simulink library "Controller_Lib"  (Simulink 8.4)
settings: Solver=ode45  StartTime=0.0  StopTime=10.0  RelTol=1e-3
values from neighbouring files (symbols this model uses):
  AC = miniMUTT_rigid_config    [UAV_config.m]    (also in UAV_modelconfig.mat = )
  TrimCondition =     [UAV_trimcondition.mat]
undefined symbols (not defined in the file or in its folder): pitch_gains, roll_gains, SampleTime
libraries: Actuator_Lib x2
settings Model: Creator=austinmurch  LastModifiedBy=brtaylor

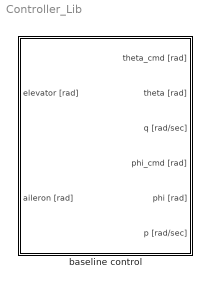
== system Controller_Lib ==
  baseline control : Subsystem  mask(Baseline Controller){pitch=0, roll=0}
      mask prompts: pitch "Pitch gains:"; roll "Roll gains:"
      mask help:
      | The "Pitch gains" parameter takes a vector input in which the first term is the
      | proportional pitch tracking gain, the second term is the integral pitch
      | tracking gain, and the third term is the pitch rate proportional gain.
      |
      | The "Roll gains" parameter takes a vector input in which the first term is the
      | proportional roll tracking gain, the second term is the integral roll tracking
      | gain, and the third term is the roll rate proportional gain.
      |
      | The yaw damper parameters take vector inputs consisting of the discrete transfer
      | function numerator and denominator coefficients.
      |
      | See Mask help for a description of the control architecture.
      mask Help:
      | This is a simple baseline controller model for the Ultrastick UAVs.
      | For the pitch axis, there is a pitch damper consisting of a proportional
      | gain on the pitch rate. The output is subtracted from the output of a
      | PI control pitch angle tracker, and the result is sent to the elevator
      | command.
      | 
      | For the roll axis, there is a roll damper consisting of a proportional
      | gain (kp_RD) on the roll rate. The output is subtracted from the output of
      | a PI control roll angle tracker, and the result is sent to the aileron
      | command.
      | 
      | For the yaw axis, there is a discrete transfer function with input yawrate,
      | and output rudder.

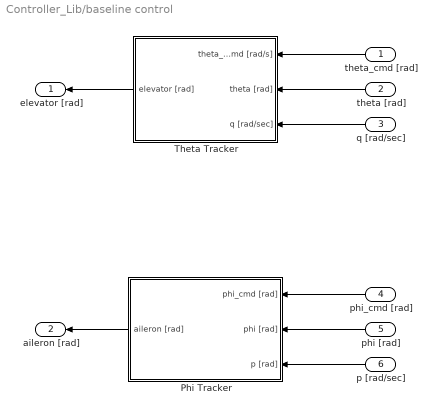
== system Controller_Lib/baseline control ==
  theta_cmd [rad] : Inport
  theta [rad] : Inport  Port=2
  q [rad/sec] : Inport  Port=3
  phi_cmd [rad] : Inport  Port=4
  phi [rad] : Inport  Port=5
  p [rad/sec] : Inport  Port=6
  Phi Tracker : Subsystem
  Theta Tracker : Subsystem
  elevator [rad] : Outport
  aileron [rad] : Outport  Port=2
  wires:
  theta_cmd [rad]/1 -> Theta Tracker/1(theta_cmd [rad/s])
  theta [rad]/1 -> Theta Tracker/2(theta [rad])
  q [rad/sec]/1 -> Theta Tracker/3(q [rad/sec])
  Theta Tracker/1(elevator [rad]) -> elevator [rad]/1
  Phi Tracker/1(aileron [rad]) -> aileron [rad]/1
  phi_cmd [rad]/1 -> Phi Tracker/1(phi_cmd [rad])
  phi [rad]/1 -> Phi Tracker/2(phi [rad])
  p [rad/sec]/1 -> Phi Tracker/3(p [rad])

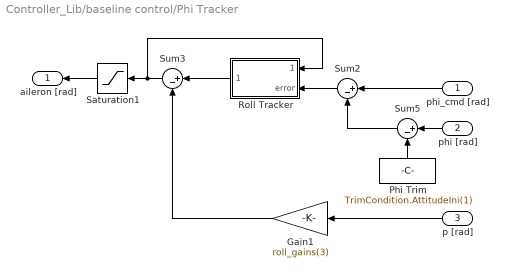
== system Controller_Lib/baseline control/Phi Tracker ==
  phi_cmd [rad] : Inport
  phi [rad] : Inport  Port=2
  p [rad] : Inport  Port=3
  Gain1 : Gain  Gain=roll_gains(3)
  Phi Trim : Constant  Value=TrimCondition.AttitudeIni(1)
  Roll Tracker : Subsystem
  Saturation1 : Saturate  UpperLimit=AC.Actuator.L2.PosLim-TrimCondition.Inputs.CtrlSurf(3)  LowerLimit=AC.Actuator.L2.NegLim-TrimCondition.Inputs.CtrlSurf(3)  SampleTime=SampleTime
  Sum2 : Sum  Inputs=|+-  SampleTime=SampleTime
  Sum3 : Sum  Inputs=|+-  SampleTime=SampleTime
  Sum5 : Sum  Inputs=|+-  SampleTime=SampleTime
  aileron [rad] : Outport
  wires:
  phi_cmd [rad]/1 -> Sum2/1
  Gain1/1 -> Sum3/2
  p [rad]/1 -> Gain1/1
  Sum3/1 -> Saturation1/1, Roll Tracker/1(aileron cmd)
  Sum2/1 -> Roll Tracker/2(error)
  Phi Trim/1 -> Sum5/2
  Sum5/1 -> Sum2/2
  phi [rad]/1 -> Sum5/1
  Saturation1/1 -> aileron [rad]/1
  Roll Tracker/1(aileron) -> Sum3/1

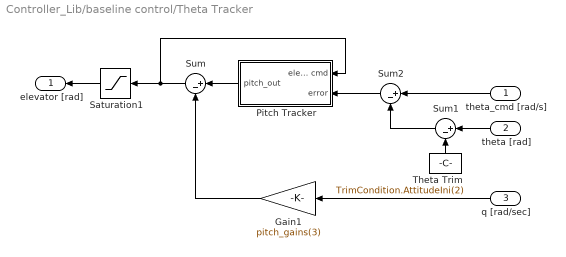
== system Controller_Lib/baseline control/Theta Tracker ==
  theta_cmd [rad/s] : Inport
  theta [rad] : Inport  Port=2
  q [rad/sec] : Inport  Port=3
  " Theta Trim" : Constant  Value=TrimCondition.AttitudeIni(2)
  Gain1 : Gain  Gain=pitch_gains(3)
  Pitch Tracker : Subsystem
  Saturation1 : Saturate  UpperLimit=AC.Actuator.L3.PosLim-TrimCondition.Inputs.CtrlSurf(1)  LowerLimit=AC.Actuator.L3.NegLim-TrimCondition.Inputs.CtrlSurf(1)  SampleTime=SampleTime
  Sum : Sum  Inputs=|+-  SampleTime=SampleTime
  Sum1 : Sum  Inputs=|+-  SampleTime=SampleTime
  Sum2 : Sum  Inputs=|+-  SampleTime=SampleTime
  elevator [rad] : Outport
  wires:
  Gain1/1 -> Sum/2
  q [rad/sec]/1 -> Gain1/1
  Sum/1 -> Saturation1/1, Pitch Tracker/1(eleveator cmd)
  Pitch Tracker/1(pitch_out) -> Sum/1
  theta_cmd [rad/s]/1 -> Sum2/1
  theta [rad]/1 -> Sum1/1
  " Theta Trim"/1 -> Sum1/2
  Sum1/1 -> Sum2/2
  Saturation1/1 -> elevator [rad]/1
  Sum2/1 -> Pitch Tracker/2(error)

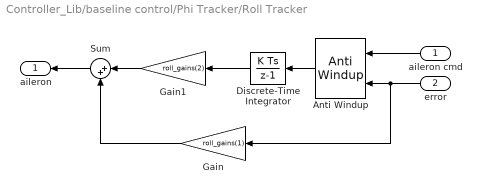
== system Controller_Lib/baseline control/Phi Tracker/Roll Tracker ==
  aileron cmd : Inport
  error : Inport  Port=2
  Anti Windup : Actuator_Lib/Anti Windup  MAX_DEF=AC.Actuator.L2.PosLim-TrimCondition.Inputs.CtrlSurf(3)  MIN_DEF=AC.Actuator.L2.NegLim-TrimCondition.Inputs.CtrlSurf(3)  gain_sign=on
  Discrete-Time Integrator : DiscreteIntegrator  SampleTime=.02
  Gain : Gain  Gain=roll_gains(1)  SampleTime=SampleTime
  Gain1 : Gain  Gain=roll_gains(2)  SampleTime=SampleTime
  Sum : Sum  Inputs=|++  SampleTime=.02
  aileron : Outport
  wires:
  Discrete-Time Integrator/1 -> Gain1/1
  Gain1/1 -> Sum/1
  Sum/1 -> aileron/1
  Gain/1 -> Sum/2
  error/1 -> Gain/1, Anti Windup/2
  aileron cmd/1 -> Anti Windup/1
  Anti Windup/1 -> Discrete-Time Integrator/1

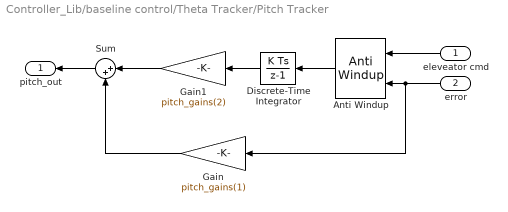
== system Controller_Lib/baseline control/Theta Tracker/Pitch Tracker ==
  eleveator cmd : Inport
  error : Inport  Port=2
  Anti Windup : Actuator_Lib/Anti Windup  MAX_DEF=AC.Actuator.L3.PosLim-TrimCondition.Inputs.CtrlSurf(1)  MIN_DEF=AC.Actuator.L3.NegLim-TrimCondition.Inputs.CtrlSurf(1)  gain_sign=off
  Discrete-Time Integrator : DiscreteIntegrator  SampleTime=.02
  Gain : Gain  Gain=pitch_gains(1)
  Gain1 : Gain  Gain=pitch_gains(2)
  Sum : Sum  Inputs=|++
  pitch_out : Outport
  wires:
  Discrete-Time Integrator/1 -> Gain1/1
  Gain1/1 -> Sum/1
  Sum/1 -> pitch_out/1
  Gain/1 -> Sum/2
  error/1 -> Gain/1, Anti Windup/2
  Anti Windup/1 -> Discrete-Time Integrator/1
  eleveator cmd/1 -> Anti Windup/1
